simulink model "open_loop_satellite_noload_2015a"  (R2015a)
settings: Solver=ode45  StartTime=0.0  StopTime=10.0  RelTol=1e-3
undefined symbols (not defined in the file): Jt, ke, km, Le, N, Re
settings Model: CovModelRefEnable=off  Creator=v.budinger  LastModifiedBy=v.budinger
settings DataIOCC: SaveFormat=Dataset
settings HardwareCC: ProdBitPerPointer=64  ProdLargestAtomicFloat=Float  ProdIntDivRoundTo=Zero  ProdEndianess=LittleEndian  ProdHWDeviceType=Specified
settings GRTTargetCC: GeneratePreprocessorConditionals=Use local settings

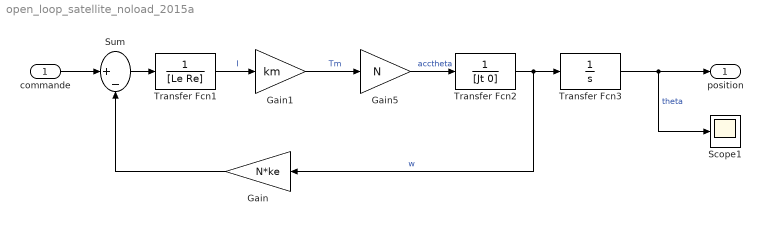
== system open_loop_satellite_noload_2015a ==
  commande : Inport
  Gain : Gain  Gain=N*ke  SaturateOnIntegerOverflow=on  OutDataTypeStr=Inherit: Same as input  ParamDataTypeStr=Inherit: Same as input
  Gain1 : Gain  Gain=km  SaturateOnIntegerOverflow=on  OutDataTypeStr=Inherit: Same as input  ParamDataTypeStr=Inherit: Same as input
  Gain5 : Gain  Gain=N  SaturateOnIntegerOverflow=on  OutDataTypeStr=Inherit: Same as input  ParamDataTypeStr=Inherit: Same as input
  Scope1 : Scope
      settings: TimeRange=auto  LimitDataPoints=on  MaxDataPoints=5000  SaveToWorkspace=off  SaveName=ScopeData  YMin=-10  YMax=10  SampleTime=-1  DataFormat=Array
  Sum : Sum  Inputs=|+-  SaturateOnIntegerOverflow=on  InputSameDT=on  OutDataTypeStr=Inherit: Same as first input
  Transfer Fcn1 : TransferFcn  Denominator=[Le Re]
  Transfer Fcn2 : TransferFcn  Denominator=[Jt 0]
  Transfer Fcn3 : TransferFcn  Denominator=[1 0]
  position : Outport
  wires:
  Sum/1 -> Transfer Fcn1/1
  Transfer Fcn1/1 -> Gain1/1  "I"
  Gain/1 -> Sum/2
  Transfer Fcn3/1 -> position/1, Scope1/1  "theta"
  commande/1 -> Sum/1
  Transfer Fcn2/1 -> Transfer Fcn3/1, Gain/1  "w"
  Gain5/1 -> Transfer Fcn2/1  "acctheta"
  Gain1/1 -> Gain5/1  "Tm"
